simulink model "invertercontrol"  (R2015a)
settings: Solver=ode45  StartTime=0.0  StopTime=0.02  RelTol=1e-3
libraries: powerlib x17, simulink x3, powerlib_meascontrol x2
settings Model: Creator=ianyl  LastModifiedBy=ianyl

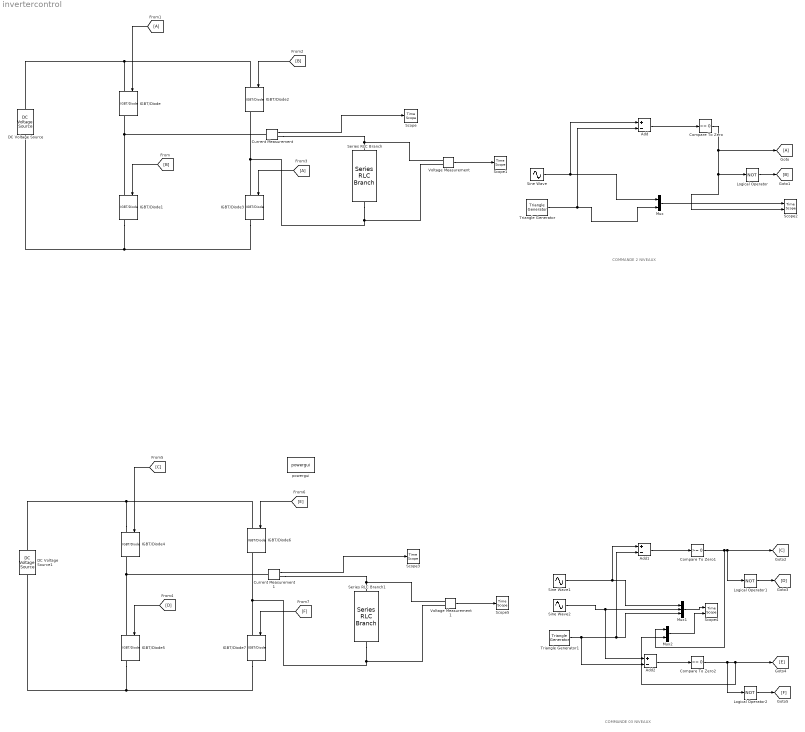
== system invertercontrol ==
  note: COMMANDE 03 NIVEAUX
  note: COMMANDE 2 NIVEAUX
  Add : Sum  Inputs=+-
  Add1 : Sum  Inputs=+-
  Add2 : Sum  Inputs=+-
  Compare To Zero : simulink/Logic and Bit Operations/Compare To Zero  relop=>=  OutDataTypeStr=boolean
  Compare To Zero1 : simulink/Logic and Bit Operations/Compare To Zero  relop=>=  OutDataTypeStr=boolean
  Compare To Zero2 : simulink/Logic and Bit Operations/Compare To Zero  relop=>=  OutDataTypeStr=boolean
  Current Measurement : powerlib/Measurements/Current Measurement  PhasorSimulation=off  OutputType=Complex  PSBequivalent=0
  Current Measurement1 : powerlib/Measurements/Current Measurement  PhasorSimulation=off  OutputType=Complex  PSBequivalent=0
  DC Voltage Source : powerlib/Electrical Sources/DC Voltage Source  Amplitude=200  Measurements=None
  DC Voltage Source1 : powerlib/Electrical Sources/DC Voltage Source  Amplitude=100  Measurements=None
  IGBT/Diode{,1..7} (8 alike) : powerlib/Power Electronics/IGBT//Diode  Ron=1e-3  Rs=1e5  Cs=inf  Measurements=on
  Logical Operator : Logic  Operator=NOT  AllPortsSameDT=off  OutDataTypeStr=boolean
  Logical Operator1 : Logic  Operator=NOT  AllPortsSameDT=off  OutDataTypeStr=boolean
  Logical Operator2 : Logic  Operator=NOT  AllPortsSameDT=off  OutDataTypeStr=boolean
  Mux : Mux  Inputs=2
  Mux1 : Mux  Inputs=3
  Mux2 : Mux  Inputs=2
  Scope{,1,3,5} (4 alike) : TimeScope
  Scope2 : TimeScope  NumInputPorts=2
  Scope4 : TimeScope  NumInputPorts=2
  Series RLC Branch : powerlib/Elements/Series RLC Branch  LConnTagsString=__new0  RConnTagsString=__new0  BranchType=RL  Resistance=100  Inductance=1e-1  SetiL0=off  InitialCurrent=0  Capacitance=1e-6  Setx0=off  InitialVoltage=0  Measurements=None
  Series RLC Branch1 : powerlib/Elements/Series RLC Branch  LConnTagsString=__new0  RConnTagsString=__new0  BranchType=RL  Resistance=100  Inductance=1e-1  SetiL0=off  InitialCurrent=0  Capacitance=1e-6  Setx0=off  InitialVoltage=0  Measurements=None
  Sine Wave : Sin  Frequency=2*pi*50  SampleTime=0
  Sine Wave1 : Sin  Frequency=2*pi*50  SampleTime=0
  Sine Wave2 : Sin  Amplitude=-1  Frequency=2*pi*50  SampleTime=0
  Triangle Generator : powerlib_meascontrol/Pulse & Signal Generators/Triangle Generator  Freq=1000  Phase=90  Ts=0
  Triangle Generator1 : powerlib_meascontrol/Pulse & Signal Generators/Triangle Generator  Freq=1500  Phase=90  Ts=0
  Voltage Measurement : powerlib/Measurements/Voltage Measurement  PhasorSimulation=off  OutputType=Complex  PSBequivalent=0
  Voltage Measurement1 : powerlib/Measurements/Voltage Measurement  PhasorSimulation=off  OutputType=Complex  PSBequivalent=0
  powergui : powerlib/powergui  Priority=1  SimulationMode=Discrete  SolverType=Tustin/Backward Euler (TBE)  SampleTime=50e-6  frequency=60  SPID=off  DisableSnubberDevices=off  DisableRonSwitches=off  DisableVfSwitches=off  SwTol=0  DisplayEquations=off  Interpol=off  methode=off  Ts=100  FunctionMessages=off  echomessages=off  HookPort=off  EnableUseOfTLC=off  x0status=blocks  frequencyindice=0  Pbase=100e6  ErrMax=1e-4  Iterations=50  UnitsV=kV  UnitsW=MW  buscounter=0  RestoreLinks=warning  ResistiveCurrentMeasurement=off  Frange=[0:2:500]  Ylog=off  Xlog=on  ShowGrid=off  save=off  variable=ZData  structure=0  ZoomFFT=off  StartTime=0.0  cycles=1  DisplayStyle=1  fundamental=60  FreqAxis=off  MaxFrequency=1000  frequencyindicesteady=1  RmsSteady=1  display=off
  wires:
  Current Measurement/1 -> Scope/1
  Voltage Measurement/1 -> Scope1/1
  Sine Wave/1 -> Add/1, Mux/1
  Triangle Generator/1 -> Add/2, Mux/2
  Mux/1 -> Scope2/1
  Add/1 -> Compare To Zero/1
  Compare To Zero/1 -> [A], Logical Operator/1, Scope2/2
  Logical Operator/1 -> [B]
  [B] -> IGBT/Diode1/1
  [A] -> IGBT/Diode/1
  [B] -> IGBT/Diode2/1
  [A] -> IGBT/Diode3/1
  Logical Operator1/1 -> [D]
  Sine Wave1/1 -> Add1/1, Mux1/1
  Sine Wave2/1 -> Add2/1, Mux1/2
  Triangle Generator1/1 -> Add2/2, Add1/2, Mux1/3
  Mux1/1 -> Scope4/1
  Add1/1 -> Compare To Zero1/1
  Add2/1 -> Compare To Zero2/1
  Compare To Zero1/1 -> Mux2/1, Logical Operator1/1, [C]
  Logical Operator2/1 -> [F]
  Compare To Zero2/1 -> Logical Operator2/1, Mux2/2, [E]
  Current Measurement1/1 -> Scope3/1
  Voltage Measurement1/1 -> Scope5/1
  [D] -> IGBT/Diode5/1
  [C] -> IGBT/Diode4/1
  [E] -> IGBT/Diode6/1
  [F] -> IGBT/Diode7/1
  Mux2/1 -> Scope4/2
  connections:
  DC Voltage Source/RConn1 -- IGBT/Diode2/LConn1 -- IGBT/Diode/LConn1
  IGBT/Diode1/RConn1 -- IGBT/Diode3/RConn1 -- DC Voltage Source/LConn1
  IGBT/Diode1/LConn1 -- Current Measurement/LConn1 -- IGBT/Diode/RConn1
  IGBT/Diode3/LConn1 -- Voltage Measurement/LConn2 -- Series RLC Branch/RConn1 -- IGBT/Diode2/RConn1
  Series RLC Branch/LConn1 -- Current Measurement/RConn1 -- Voltage Measurement/LConn1
  IGBT/Diode4/LConn1 -- DC Voltage Source1/RConn1 -- IGBT/Diode6/LConn1
  DC Voltage Source1/LConn1 -- IGBT/Diode5/RConn1 -- IGBT/Diode7/RConn1
  IGBT/Diode5/LConn1 -- Current Measurement1/LConn1 -- IGBT/Diode4/RConn1
  IGBT/Diode7/LConn1 -- Voltage Measurement1/LConn2 -- Series RLC Branch1/RConn1 -- IGBT/Diode6/RConn1
  Series RLC Branch1/LConn1 -- Current Measurement1/RConn1 -- Voltage Measurement1/LConn1
